simulink model "asg2_3k04"  (R2019a)
settings: Solver=FixedStepAuto  StartTime=0.0  StopTime=100  FixedStep=1E-3  RelTol=1e-3
undefined symbols (not defined in the file): D0, D1, D10, D11, D12, D13, D2, D3, D4, D5, D6, D7, D8, D9, PTA0, PTA1, PTA2, PTB23, PTB9, PTC16, PTC17, PTC2, PTC3, PTC4, PTD0, PTD1, PTD2, PTD3
libraries: frdmk64flib x21
settings Model: ExtModeTrigDuration=5  Creator=junbo  LastModifiedBy=Junbo Huang
settings OptimizationCC: EnhancedBackFolding=on  PassReuseOutputArgsAs=Individual arguments  MaxStackSize=64  OptimizeBlockOrder=speed  DifferentSizesBufferReuse=on  OptimizationCustomize=off
settings DebuggingCC: ParameterTunabilityLossMsg=error
settings HardwareCC: ProdBitPerPointer=32  ProdBitPerSizeT=32  ProdBitPerPtrDiffT=32  ProdLargestAtomicInteger=Long  ProdLargestAtomicFloat=Double  ProdWordSize=32  ProdHWDeviceType=ARM Compatible->ARM Cortex
settings SFSimCC: MATLABDynamicMemAlloc=off
settings RTWCC: SystemTargetFile=ert.tlc  HardwareBoard=NXP FRDM-K64F  TLCOptions="-aInlineSetEventsForThisBaseRateFcn=TLC_FALSE -aSuppressMultiTaskScheduler=TLC_FALSE  -aRateBasedStepFcn=0"  TemplateMakefile=ert_default_tmf  GenerateReport=on  Toolchain=GNU Tools for ARM Embedded Processors  IncludeHyperlinkInReport=on  LaunchReport=on  GenerateTraceInfo=on  GenerateTraceReport=on  GenerateTraceReportSl=on  GenerateTraceReportSf=on  GenerateTraceReportEml=on
settings CodeAppCC: ForceParamTrailComments=on  IgnoreCustomStorageClasses=off  OperatorAnnotations=on  SimulinkDataObjDesc=on  SFDataObjDesc=on  InsertBlockDesc=on
settings ERTTargetCC: SupportContinuousTime=on

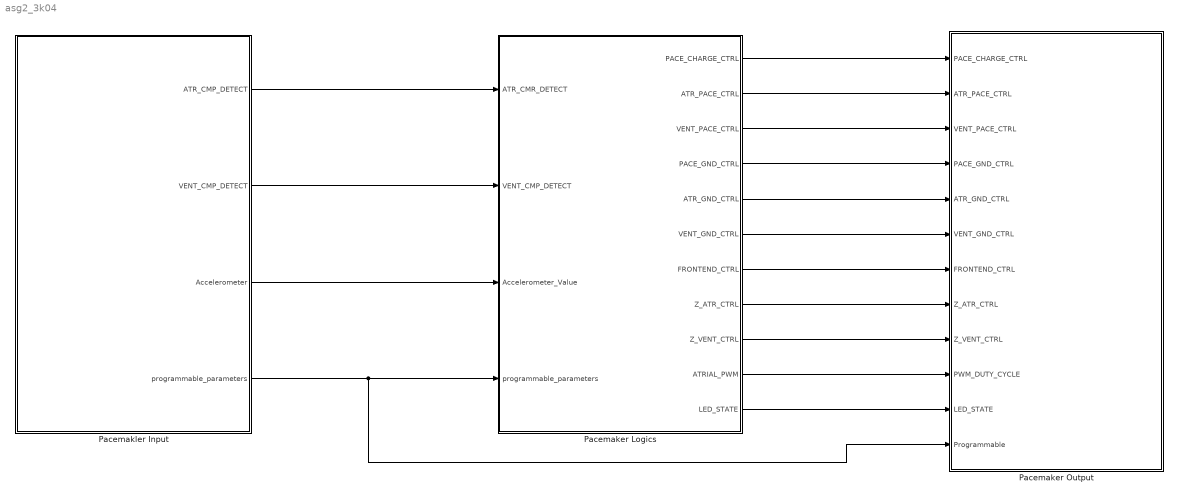
== system asg2_3k04 ==
  Pacemaker Logics : Subsystem
  Pacemaker Output : Subsystem
  Pacemakler Input : Subsystem
  wires:
  Pacemakler Input/3("Accelerometer ") -> Pacemaker Logics/3(Accelerometer_Value)
  Pacemaker Logics/11(LED_STATE) -> Pacemaker Output/11(LED_STATE)
  Pacemaker Logics/10(ATRIAL_PWM) -> Pacemaker Output/10(PWM_DUTY_CYCLE)
  Pacemaker Logics/4(PACE_GND_CTRL) -> Pacemaker Output/4(PACE_GND_CTRL)
  Pacemakler Input/1(ATR_CMP_DETECT) -> Pacemaker Logics/1(ATR_CMR_DETECT)
  Pacemaker Logics/6(VENT_GND_CTRL) -> Pacemaker Output/6(VENT_GND_CTRL)
  Pacemaker Logics/9(Z_VENT_CTRL) -> Pacemaker Output/9(Z_VENT_CTRL)
  Pacemaker Logics/8(Z_ATR_CTRL) -> Pacemaker Output/8(Z_ATR_CTRL)
  Pacemaker Logics/2(ATR_PACE_CTRL) -> Pacemaker Output/2(ATR_PACE_CTRL)
  Pacemaker Logics/3(VENT_PACE_CTRL) -> Pacemaker Output/3(VENT_PACE_CTRL)
  Pacemakler Input/2(VENT_CMP_DETECT) -> Pacemaker Logics/2(VENT_CMP_DETECT)
  Pacemaker Logics/5(ATR_GND_CTRL) -> Pacemaker Output/5(ATR_GND_CTRL)
  Pacemaker Logics/1(PACE_CHARGE_CTRL) -> Pacemaker Output/1(PACE_CHARGE_CTRL)
  Pacemakler Input/4(programmable_parameters) -> Pacemaker Output/12("Programmable "), Pacemaker Logics/4(programmable_parameters)
  Pacemaker Logics/7(FRONTEND_CTRL) -> Pacemaker Output/7(FRONTEND_CTRL)

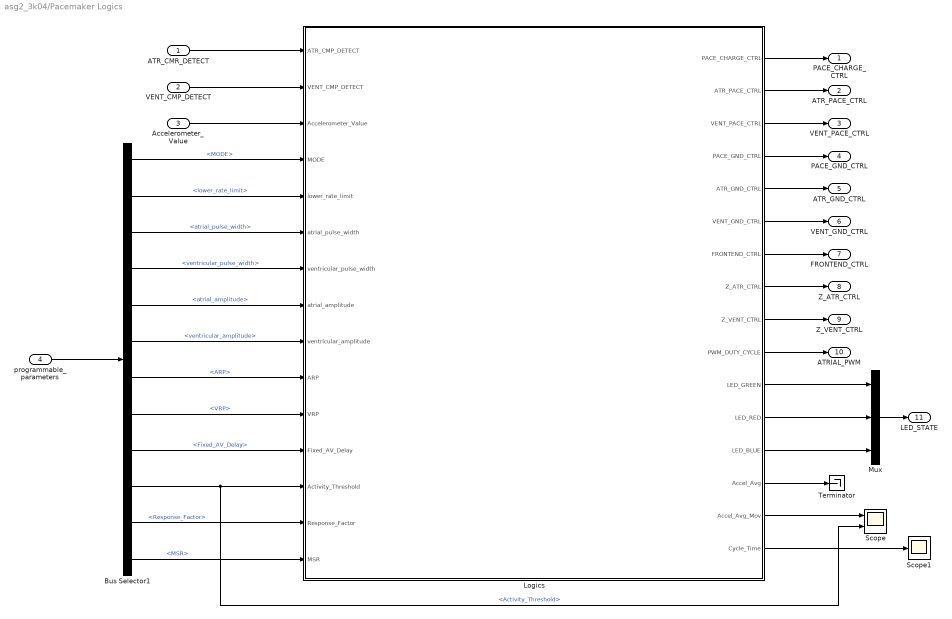
== system asg2_3k04/Pacemaker Logics ==
  ATR_CMR_DETECT : Inport
  VENT_CMP_DETECT : Inport  Port=2
  Accelerometer_Value : Inport  Port=3
  programmable_parameters : Inport  Port=4
  Bus Selector1 : BusSelector  OutputSignals=MODE,lower_rate_limit,atrial_pulse_width,ventricular_pulse_width,atrial_amplitude,ventricular_amplitude,ARP,VRP,Fixed_AV_Delay,Activity_Threshold,Response_Factor,MSR
  Logics : Stateflow chart  TreatAsAtomicUnit=on
  Mux : Mux  Inputs=3
  Scope : Scope  NumInputPorts=2
  Scope1 : Scope
  Terminator : Terminator
  PACE_CHARGE_CTRL : Outport
  ATR_PACE_CTRL : Outport  Port=2
  VENT_PACE_CTRL : Outport  Port=3
  PACE_GND_CTRL : Outport  Port=4
  ATR_GND_CTRL : Outport  Port=5
  VENT_GND_CTRL : Outport  Port=6
  FRONTEND_CTRL : Outport  Port=7
  Z_ATR_CTRL : Outport  Port=8
  Z_VENT_CTRL : Outport  Port=9
  ATRIAL_PWM : Outport  Port=10
  LED_STATE : Outport  Port=11
  wires:
  Logics/1(PACE_CHARGE_CTRL) -> PACE_CHARGE_CTRL/1
  Bus Selector1/7 -> Logics/10(ARP)  "<ARP>"
  Bus Selector1/8 -> Logics/11(VRP)  "<VRP>"
  Bus Selector1/4 -> Logics/7(ventricular_pulse_width)  "<ventricular_pulse_width>"
  Logics/2(ATR_PACE_CTRL) -> ATR_PACE_CTRL/1
  Bus Selector1/6 -> Logics/9(ventricular_amplitude)  "<ventricular_amplitude>"
  Bus Selector1/5 -> Logics/8(atrial_amplitude)  "<atrial_amplitude>"
  Bus Selector1/2 -> Logics/5(lower_rate_limit)  "<lower_rate_limit>"
  Logics/9(Z_VENT_CTRL) -> Z_VENT_CTRL/1
  Logics/8(Z_ATR_CTRL) -> Z_ATR_CTRL/1
  Logics/7(FRONTEND_CTRL) -> FRONTEND_CTRL/1
  programmable_parameters/1 -> Bus Selector1/1
  Bus Selector1/1 -> Logics/4(MODE)  "<MODE>"
  Bus Selector1/3 -> Logics/6(atrial_pulse_width)  "<atrial_pulse_width>"
  VENT_CMP_DETECT/1 -> Logics/2(VENT_CMP_DETECT)
  Logics/4(PACE_GND_CTRL) -> PACE_GND_CTRL/1
  Logics/5(ATR_GND_CTRL) -> ATR_GND_CTRL/1
  Logics/6(VENT_GND_CTRL) -> VENT_GND_CTRL/1
  ATR_CMR_DETECT/1 -> Logics/1(ATR_CMP_DETECT)
  Logics/3(VENT_PACE_CTRL) -> VENT_PACE_CTRL/1
  Logics/10(PWM_DUTY_CYCLE) -> ATRIAL_PWM/1
  Bus Selector1/9 -> Logics/12(Fixed_AV_Delay)  "<Fixed_AV_Delay>"
  Accelerometer_Value/1 -> Logics/3(Accelerometer_Value)
  Logics/11(LED_GREEN) -> Mux/1
  Logics/12(LED_RED) -> Mux/2
  Logics/13(LED_BLUE) -> Mux/3
  Mux/1 -> LED_STATE/1
  Bus Selector1/10 -> Scope/2, Logics/13(Activity_Threshold)  "<Activity_Threshold>"
  Bus Selector1/11 -> Logics/14(Response_Factor)  "<Response_Factor>"
  Bus Selector1/12 -> Logics/15(MSR)  "<MSR>"
  Logics/14(Accel_Avg) -> Terminator/1
  Logics/15(Accel_Avg_Mov) -> Scope/1
  Logics/16(Cycle_Time) -> Scope1/1

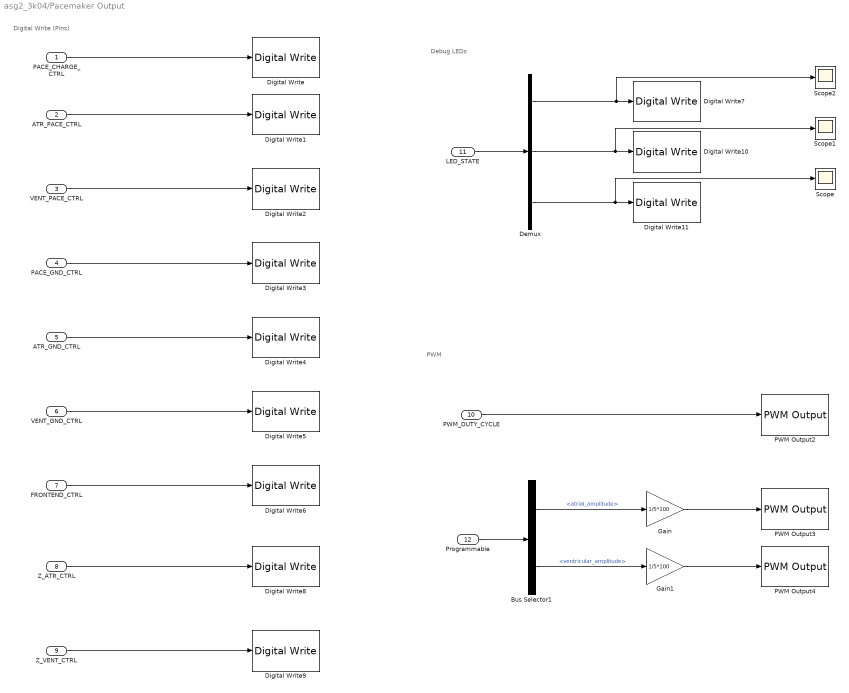
== system asg2_3k04/Pacemaker Output ==
  note: Digital Write (Pins)
  note: PWM
  note: Debug LEDs
  PACE_CHARGE_CTRL : Inport
  ATR_PACE_CTRL : Inport  Port=2
  VENT_PACE_CTRL : Inport  Port=3
  PACE_GND_CTRL : Inport  Port=4
  ATR_GND_CTRL : Inport  Port=5
  VENT_GND_CTRL : Inport  Port=6
  FRONTEND_CTRL : Inport  Port=7
  Z_ATR_CTRL : Inport  Port=8
  Z_VENT_CTRL : Inport  Port=9
  PWM_DUTY_CYCLE : Inport  Port=10
  LED_STATE : Inport  Port=11
  "Programmable " : Inport  Port=12
  Bus Selector1 : BusSelector  OutputSignals=atrial_amplitude,ventricular_amplitude
  Demux : Demux  Outputs=3
  Digital Write : frdmk64flib/Digital Write  Whichpin=PTB9 (D2)
      settings: SourceProductName=Simulink Coder Support Package for NXP FRDM-K64F Board
  Digital Write1 : frdmk64flib/Digital Write  Whichpin=PTA0 (D8)
      settings: SourceProductName=Simulink Coder Support Package for NXP FRDM-K64F Board
  Digital Write10 : frdmk64flib/Digital Write  Whichpin=RED_LED
      settings: SourceProductName=Simulink Coder Support Package for NXP FRDM-K64F Board
  Digital Write11 : frdmk64flib/Digital Write  Whichpin=BLUE_LED
      settings: SourceProductName=Simulink Coder Support Package for NXP FRDM-K64F Board
  Digital Write2 : frdmk64flib/Digital Write  Whichpin=PTC4 (D9)
      settings: SourceProductName=Simulink Coder Support Package for NXP FRDM-K64F Board
  Digital Write3 : frdmk64flib/Digital Write  Whichpin=PTD0 (D10)
      settings: SourceProductName=Simulink Coder Support Package for NXP FRDM-K64F Board
  Digital Write4 : frdmk64flib/Digital Write  Whichpin=PTD2 (D11)
      settings: SourceProductName=Simulink Coder Support Package for NXP FRDM-K64F Board
  Digital Write5 : frdmk64flib/Digital Write  Whichpin=PTD3 (D12)
      settings: SourceProductName=Simulink Coder Support Package for NXP FRDM-K64F Board
  Digital Write6 : frdmk64flib/Digital Write  Whichpin=PTD1 (D13)
      settings: SourceProductName=Simulink Coder Support Package for NXP FRDM-K64F Board
  Digital Write7 : frdmk64flib/Digital Write  Whichpin=GREEN_LED
      settings: SourceProductName=Simulink Coder Support Package for NXP FRDM-K64F Board
  Digital Write8 : frdmk64flib/Digital Write  Whichpin=PTB23 (D4)
      settings: SourceProductName=Simulink Coder Support Package for NXP FRDM-K64F Board
  Digital Write9 : frdmk64flib/Digital Write  Whichpin=PTC3 (D7)
      settings: SourceProductName=Simulink Coder Support Package for NXP FRDM-K64F Board
  Gain : Gain  Gain=1/5*100
  Gain1 : Gain  Gain=1/5*100
  PWM Output2 : frdmk64flib/PWM Output  Whichpin=PTA2 (D5)  InitialFrequency=2000  InitialDutyCycle=0
      settings: SourceProductName=Simulink Coder Support Package for NXP FRDM-K64F Board
  PWM Output3 : frdmk64flib/PWM Output  Whichpin=PTC2 (D6)  InitialFrequency=2000  InitialDutyCycle=0
      settings: SourceProductName=Simulink Coder Support Package for NXP FRDM-K64F Board
  PWM Output4 : frdmk64flib/PWM Output  Whichpin=PTA1 (D3)  InitialFrequency=2000  InitialDutyCycle=0
      settings: SourceProductName=Simulink Coder Support Package for NXP FRDM-K64F Board
  Scope : Scope
  Scope1 : Scope
  Scope2 : Scope
  wires:
  PACE_CHARGE_CTRL/1 -> Digital Write/1
  FRONTEND_CTRL/1 -> Digital Write6/1
  ATR_PACE_CTRL/1 -> Digital Write1/1
  VENT_PACE_CTRL/1 -> Digital Write2/1
  PACE_GND_CTRL/1 -> Digital Write3/1
  ATR_GND_CTRL/1 -> Digital Write4/1
  VENT_GND_CTRL/1 -> Digital Write5/1
  Z_ATR_CTRL/1 -> Digital Write8/1
  Z_VENT_CTRL/1 -> Digital Write9/1
  Bus Selector1/1 -> Gain/1  "<atrial_amplitude>"
  Bus Selector1/2 -> Gain1/1  "<ventricular_amplitude>"
  "Programmable "/1 -> Bus Selector1/1
  PWM_DUTY_CYCLE/1 -> PWM Output2/1
  Gain/1 -> PWM Output3/1
  Gain1/1 -> PWM Output4/1
  Demux/3 -> Scope/1, Digital Write11/1
  LED_STATE/1 -> Demux/1
  Demux/1 -> Scope2/1, Digital Write7/1
  Demux/2 -> Scope1/1, Digital Write10/1

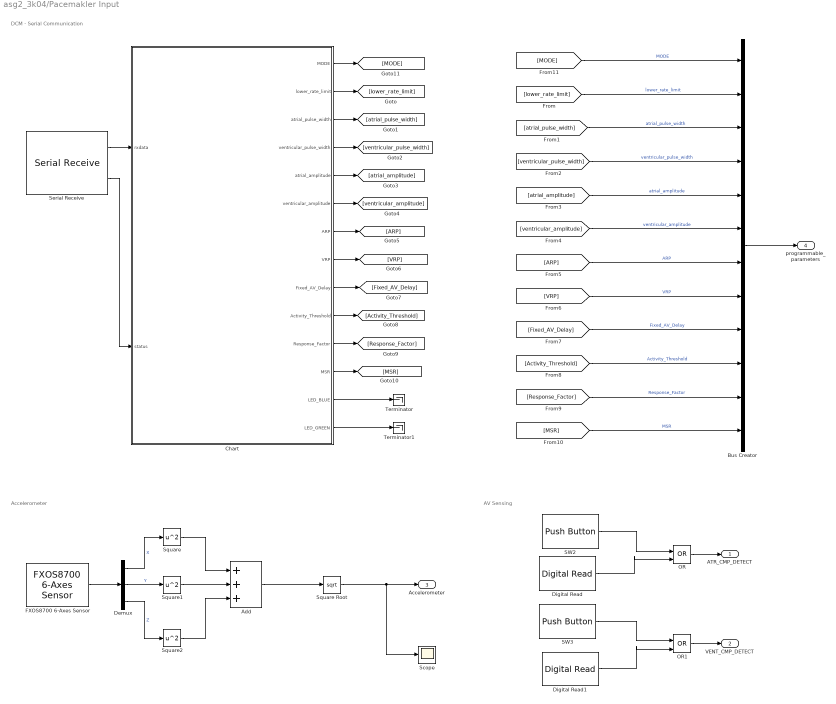
== system asg2_3k04/Pacemakler Input ==
  note: DCM - Serial Communication
  note: Accelerometer
  note: AV Sensing
  Add : Sum  Inputs=+++
  Bus Creator : BusCreator  Inputs=12
  Chart : Stateflow chart  BlockKeywords=__PRM__SERIALIZED__DATA__:Stateflow Chart,Stateflow Diagram  TreatAsAtomicUnit=on
  Demux : Demux  Outputs=3
  Digital Read : frdmk64flib/Digital Read  Whichpin=PTC16 (D0)  SampleTime=-1
      settings: SourceProductName=Simulink Coder Support Package for NXP FRDM-K64F Board
  Digital Read1 : frdmk64flib/Digital Read  Whichpin=PTC17 (D1)  SampleTime=-1
      settings: SourceProductName=Simulink Coder Support Package for NXP FRDM-K64F Board
  FXOS8700 6-Axes Sensor : frdmk64flib/FXOS8700 6-Axes Sensor  Activesensor=Accelerometer only  ODR=800Hz  HybridODR=400Hz  Accelfullrange=-4g to +4g  SampleTime=-1
      settings: SourceProductName=Simulink Coder Support Package for NXP FRDM-K64F Board
  OR : Logic  Operator=OR  IconShape=distinctive  AllPortsSameDT=off  OutDataTypeStr=boolean
  OR1 : Logic  Operator=OR  IconShape=distinctive  AllPortsSameDT=off  OutDataTypeStr=boolean
  SW2 : frdmk64flib/Push Button  Whichswitch=SW2  SampleTime1=-1
      settings: SourceProductName=Simulink Coder Support Package for NXP FRDM-K64F Board
  SW3 : frdmk64flib/Push Button  Whichswitch=SW3  SampleTime1=-1
      settings: SourceProductName=Simulink Coder Support Package for NXP FRDM-K64F Board
  Scope : Scope
  Serial Receive : frdmk64flib/Serial Receive  SCIModule=0  Baudrate=uint32(9600)  Parity=None  StopBits=1  HardwareFlowControl=None  ByteOrder=LittleEndian  DataType=uint8  DataLength=52  BlockingMode=off  OutputStatus=on  SampleTime=-1
      settings: SourceProductName=Simulink Coder Support Package for NXP FRDM-K64F Board
  Square : Math  Operator=square  SaturateOnIntegerOverflow=on
  Square Root : Sqrt  SaturateOnIntegerOverflow=on
  Square1 : Math  Operator=square  SaturateOnIntegerOverflow=on
  Square2 : Math  Operator=square  SaturateOnIntegerOverflow=on
  Terminator : Terminator
  Terminator1 : Terminator
  ATR_CMP_DETECT : Outport
  VENT_CMP_DETECT : Outport  Port=2
  "Accelerometer " : Outport  Port=3
  programmable_parameters : Outport  Port=4
  wires:
  OR/1 -> ATR_CMP_DETECT/1
  SW2/1 -> OR/1
  OR1/1 -> VENT_CMP_DETECT/1
  SW3/1 -> OR1/1
  Bus Creator/1 -> programmable_parameters/1
  [lower_rate_limit] -> Bus Creator/2  "lower_rate_limit"
  [atrial_pulse_width] -> Bus Creator/3  "atrial_pulse_width"
  [ventricular_pulse_width] -> Bus Creator/4  "ventricular_pulse_width"
  [VRP] -> Bus Creator/8  "VRP"
  [ARP] -> Bus Creator/7  "ARP"
  [atrial_amplitude] -> Bus Creator/5  "atrial_amplitude"
  [ventricular_amplitude] -> Bus Creator/6  "ventricular_amplitude"
  [Fixed_AV_Delay] -> Bus Creator/9  "Fixed_AV_Delay"
  FXOS8700 6-Axes Sensor/1 -> Demux/1
  Demux/1 -> Square/1  "X"
  Demux/2 -> Square1/1  "Y"
  Demux/3 -> Square2/1  "Z"
  Square/1 -> Add/1
  Square1/1 -> Add/2
  Square2/1 -> Add/3
  Add/1 -> Square Root/1
  [Activity_Threshold] -> Bus Creator/10  "Activity_Threshold"
  [Response_Factor] -> Bus Creator/11  "Response_Factor"
  [MSR] -> Bus Creator/12  "MSR"
  Square Root/1 -> Scope/1, "Accelerometer "/1
  [MODE] -> Bus Creator/1  "MODE"
  Chart/2(lower_rate_limit) -> [lower_rate_limit]
  Chart/3(atrial_pulse_width) -> [atrial_pulse_width]
  Chart/4(ventricular_pulse_width) -> [ventricular_pulse_width]
  Chart/5(atrial_amplitude) -> [atrial_amplitude]
  Chart/6(ventricular_amplitude) -> [ventricular_amplitude]
  Chart/7(ARP) -> [ARP]
  Chart/8(VRP) -> [VRP]
  Chart/9(Fixed_AV_Delay) -> [Fixed_AV_Delay]
  Chart/10(Activity_Threshold) -> [Activity_Threshold]
  Chart/11(Response_Factor) -> [Response_Factor]
  Chart/12(MSR) -> [MSR]
  Chart/1(MODE) -> [MODE]
  Chart/13(LED_BLUE) -> Terminator/1
  Chart/14(LED_GREEN) -> Terminator1/1
  Digital Read1/1 -> OR1/2
  Digital Read/1 -> OR/2
  Serial Receive/1 -> Chart/1(rxdata)
  Serial Receive/2 -> Chart/2(status)

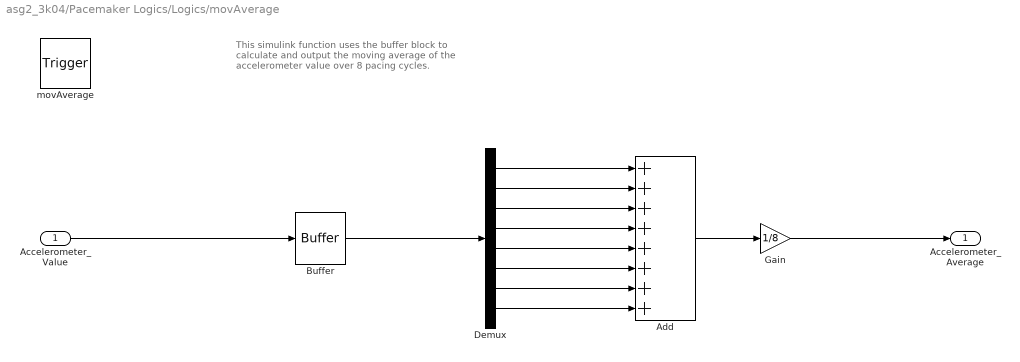
== system asg2_3k04/Pacemaker Logics/Logics/movAverage ==
  note: This simulink function uses the buffer block to calculate and output the moving average of the accelerometer value over 8 pacing cycles.
  Accelerometer_Value : Inport  OutDataTypeStr=double  PortDimensions=1
  "movAverage " : TriggerPort  TriggerType=function-call  VariantControl=(inherit)
      settings: CopyFcn=Stateflow.SLINSF.SimulinkMan.removeBlockPreDeleteFcn  PreDeleteFcn=Stateflow.SLINSF.SimulinkMan.unsafePredeleteFcn
  Add : Sum  Inputs=++++++++
  Buffer : Buffer  N=8  V=7  ic=1  OutputFrames=off
  Demux : Demux  Outputs=8
  Gain : Gain  Gain=1/8
  Accelerometer_Average : Outport  PortDimensions=1
  wires:
  Accelerometer_Value/1 -> Buffer/1
  Buffer/1 -> Demux/1
  Demux/1 -> Add/1
  Demux/2 -> Add/2
  Demux/3 -> Add/3
  Demux/4 -> Add/4
  Demux/5 -> Add/5
  Add/1 -> Gain/1
  Gain/1 -> Accelerometer_Average/1
  Demux/6 -> Add/6
  Demux/7 -> Add/7
  Demux/8 -> Add/8

== stateflow chart asg2_3k04/Pacemakler Input/Chart ==
  note: Data are unpacked and written to
      | the simulink variables as inputs.
  state Update
    entry:
    LED_BLUE = 0;
    LED_GREEN = 0;
    MODE = typecast(rxdata(3:4), 'uint16');
    %%%%
    lower_rate_limit = typecast(rxdata(5:8), 'single');
    %upper_rate_limit = typecast(rxdata(9:12), 'single');
    MSR = typecast(rxdata(13:16), 'single');
    Fixed_AV_Delay = typecast(rxdata(17:20), 'single');
    %%%%
    atrial_amplitude = typecast(rxdata(21:24), 'single');
    ventricular_amplitude = typecast(rxdata(25:28), 'single');
    atrial_pulse_width = typecast(rxdata(29:32), 'single');
    ventricular_pulse_width = typecast(rxdata(33:36), 'single');
    %%%%
    VRP = typecast(rxdata(37:40), 'single');
    ARP = typecast(rxdata(41:44), 'single');
    Activity_Threshold = typecast(rxdata(45:48), 'single');
    Response_Factor = typecast(rxdata(49:52), 'single');
  state Init
    entry:
    MODE= 5;
    lower_rate_limit=60;
    atrial_pulse_width=20;
    ventricular_pulse_width=20;
    atrial_amplitude=3;
    ventricular_amplitude=3;
    ARP=150;
    VRP=150;
    Fixed_AV_Delay=20;
    Activity_Threshold=1.5;
    Response_Factor=1;
    MSR = 120;
    LED_GREEN = 0;
    LED_BLUE = 0;
    %%%%%%Initialize Parameters%%%%%%%%
  state StandBy
    entry:
    LED_BLUE = 0;
    LED_GREEN = 0;
  note: Check if serial
      | com succeed
  note: Check the first byte of
      | Serial Data
  note: We set the first byte to 1 in
      | DCM and an acknowledgement
      | for the begin of packed serial data
  (default) -> Init
  Update -> StandBy : after(500, msec)
  (junction 42) -> StandBy [order 2]
  Init -> StandBy
  StandBy -> (junction 42) : [status == 0]
  (junction 42) -> Update [order 1] : [rxdata(1) == hex2dec('1') ]
  data: MODE output uint16; rxdata input uint8; status input uint8; lower_rate_limit output single; atrial_pulse_width output single; ventricular_pulse_width output single; atrial_amplitude output single; ventricular_amplitude output single; ARP output single; VRP output single; Fixed_AV_Delay output single; Activity_Threshold output single; Response_Factor output single; MSR output single; LED_BLUE output uint8; LED_GREEN output uint8

== stateflow chart asg2_3k04/Pacemaker Logics/Logics ==
  state VOO_MODE
    note: Charge up C22 and discharge C21 to ground
    note: Discharge C22 to C21 which charge up C21
    state VOO_CHARGE
      entry:
      PACE_CHARGE_CTRL = true;
      VENT_PACE_CTRL = false;
      VENT_GND_CTRL = true;
      PACE_GND_CTRL = true;
      Z_ATR_CTRL = false;
      Z_VENT_CTRL = false;
      Cycle_Time = (60/lower_rate_limit)*1000;
      LED_GREEN = 0;
    state VOO_PACE
      entry:
      PACE_CHARGE_CTRL = false;
      VENT_PACE_CTRL = true;
      VENT_GND_CTRL = false;
      PACE_GND_CTRL = true;
      Z_ATR_CTRL = false;
      Z_VENT_CTRL = false;
      PWM_DUTY_CYCLE = (ventricular_amplitude/5)*100;
      LED_GREEN = 1;
    VOO_MODE.VOO_CHARGE -> VOO_MODE.VOO_PACE [order 2] : after(Cycle_Time - ventricular_pulse_width,msec)
    VOO_MODE.VOO_PACE -> VOO_MODE.VOO_CHARGE : after(ventricular_pulse_width,msec)
  state VOOR_MODE
    state PACE [parallel]
      settings: executionOrder=1
      note: Charge up C22 and discharge C21 to ground
      note: Discharge C22 to C21 which charge up C21
      state VOO_CHARGE
        entry:
        PACE_CHARGE_CTRL = true;
        VENT_PACE_CTRL = false;
        VENT_GND_CTRL = true;
        PACE_GND_CTRL = true;
        Z_ATR_CTRL = false;
        Z_VENT_CTRL = false;
        LED_GREEN = 0;
        Accel_Avg_Mov = movAverage(Accel_Avg);
        Cycle_Time = rateConversion(lower_rate_limit, MSR, Response_Factor, Activity_Threshold, Accel_Avg_Mov);
      state VOO_PACE
        entry:
        PACE_CHARGE_CTRL = false;
        VENT_PACE_CTRL = true;
        VENT_GND_CTRL = false;
        PACE_GND_CTRL = true;
        Z_ATR_CTRL = false;
        Z_VENT_CTRL = false;
        PWM_DUTY_CYCLE = (ventricular_amplitude/5)*100;
        LED_GREEN = 1;
      VOOR_MODE.PACE.VOO_CHARGE -> VOOR_MODE.PACE.VOO_PACE [order 1] : after(Cycle_Time - ventricular_pulse_width,msec)
      (default) -> VOOR_MODE.PACE.VOO_CHARGE
      VOOR_MODE.PACE.VOO_PACE -> VOOR_MODE.PACE.VOO_CHARGE : after(ventricular_pulse_width,msec)
    state RateAdaptive [parallel]
      settings: executionOrder=2
      state Update_Acc_Avg
        entry:
        [Accel_Avg, Cycle_Counter] = average(Accel_Val_Vec, Cycle_Counter);
      state Store_Acc_Val
        entry:
        [Accel_Val_Vec, Cycle_Counter] = storeSamples(Accelerometer_Value, Accel_Val_Vec, Cycle_Counter);
      VOOR_MODE.RateAdaptive.Store_Acc_Val -> VOOR_MODE.RateAdaptive.Update_Acc_Avg [order 1] : [Cycle_Counter >= 500]
      VOOR_MODE.RateAdaptive.Update_Acc_Avg -> VOOR_MODE.RateAdaptive.Store_Acc_Val
      (default) -> VOOR_MODE.RateAdaptive.Store_Acc_Val
      VOOR_MODE.RateAdaptive.Store_Acc_Val -> VOOR_MODE.RateAdaptive.Store_Acc_Val [order 2]
  state Accelerometer_Average = movAverage(Accelerometer_Value) [function]
  note: Starting state, open all the switchs for safety
  state Initialize
    entry:
    Cycle_Time = (60/lower_rate_limit)*1000;
    Accel_Val_Vec = ones(500,1);
    Accel_Avg = 1;
    Accel_Avg_Mov = 1;
    Cycle_Counter = 0;
  note: VOO Mode
  state AOO_MODE
    note: Charge up C22 and discharge C21 to ground
    note: Discharge C22 to C21 which charge up C21
    state AOO_CHARGE
      entry:
      PACE_CHARGE_CTRL = true;
      %charge C22
      ATR_PACE_CTRL = false;
      ATR_GND_CTRL = true;
      PACE_GND_CTRL = true;
      %discharge C21
      Z_ATR_CTRL = false;
      Z_VENT_CTRL = false;
      Cycle_Time = (60/lower_rate_limit)*1000;
      LED_RED = 0;
    state AOO_PACE
      entry:
      PACE_CHARGE_CTRL = false;
      PACE_GND_CTRL = true; %charge C21
      ATR_PACE_CTRL = true; %discharge C22
      ATR_GND_CTRL = false;
      Z_ATR_CTRL = false;
      Z_VENT_CTRL = false;
      PWM_DUTY_CYCLE = (atrial_amplitude/5)*100;
      %set PWM duty cycle based on input amplitude
      LED_RED = 1;
    note: Lower rate limit is converted to period of cycle
    note: Pace for the period specified by pulse width
    AOO_MODE.AOO_CHARGE -> AOO_MODE.AOO_PACE [order 1] : after(Cycle_Time - atrial_pulse_width,msec)
    AOO_MODE.AOO_PACE -> AOO_MODE.AOO_CHARGE : after(atrial_pulse_width,msec)
  state AOOR_MODE
    state Pace [parallel]
      settings: executionOrder=1
      note: Charge up C22 and discharge C21 to ground
      note: Discharge C22 to C21 which charge up C21
      state AOO_CHARGE
        entry:
        PACE_CHARGE_CTRL = true;
        %charge C22
        ATR_PACE_CTRL = false;
        ATR_GND_CTRL = true;
        PACE_GND_CTRL = true;
        %discharge C21
        Z_ATR_CTRL = false;
        Z_VENT_CTRL = false;
        LED_RED = 0;
        Accel_Avg_Mov = movAverage(Accel_Avg);
        Cycle_Time = rateConversion(lower_rate_limit, MSR, Response_Factor, Activity_Threshold, Accel_Avg_Mov);
      state AOO_PACE
        entry:
        PACE_CHARGE_CTRL = false;
        PACE_GND_CTRL = true; %charge C21
        ATR_PACE_CTRL = true; %discharge C22
        ATR_GND_CTRL = false;
        Z_ATR_CTRL = false;
        Z_VENT_CTRL = false;
        PWM_DUTY_CYCLE = (atrial_amplitude/5)*100;
        LED_RED = 1
        %set PWM duty cycle based on input amplitude
      note: Lower rate limit is converted to period of cycle
      note: Pace for the period specified by pulse width
      AOOR_MODE.Pace.AOO_CHARGE -> AOOR_MODE.Pace.AOO_PACE [order 1] : after(Cycle_Time - atrial_pulse_width,msec)
      (default) -> AOOR_MODE.Pace.AOO_CHARGE
      AOOR_MODE.Pace.AOO_PACE -> AOOR_MODE.Pace.AOO_CHARGE : after(atrial_pulse_width,msec)
    state RateAdaptive [parallel]
      settings: executionOrder=2
      state Update_Acc_Avg
        entry:
        [Accel_Avg, Cycle_Counter] = average(Accel_Val_Vec, Cycle_Counter);
      state Store_Acc_Val
        entry:
        [Accel_Val_Vec, Cycle_Counter] = storeSamples(Accelerometer_Value, Accel_Val_Vec, Cycle_Counter);
      AOOR_MODE.RateAdaptive.Store_Acc_Val -> AOOR_MODE.RateAdaptive.Update_Acc_Avg [order 1] : [Cycle_Counter >= 500]
      AOOR_MODE.RateAdaptive.Update_Acc_Avg -> AOOR_MODE.RateAdaptive.Store_Acc_Val
      (default) -> AOOR_MODE.RateAdaptive.Store_Acc_Val
      AOOR_MODE.RateAdaptive.Store_Acc_Val -> AOOR_MODE.RateAdaptive.Store_Acc_Val [order 2]
  state MAIN
    entry:
    PACE_CHARGE_CTRL = false;
    VENT_PACE_CTRL = false;
    ATR_PACE_CTRL = false;
    VENT_GND_CTRL = false;
    ATR_GND_CTRL = false;
    PACE_GND_CTRL = false;
    FRONTEND_CTRL = false;
    Z_ATR_CTRL = false;
    Z_VENT_CTRL = false;
    %%% Initialize LEDs
    LED_GREEN = 0;
    LED_RED = 0;
    LED_BLUE = 0;
  note: AOO Mode
  note: MODE
      | Mode Name
      |
      | 0
      | VOO
      |
      | 1
      | AOO
      |
      | 2
      | VVI
      |
      | 3
      | AAI
      |
      | 4
      | DOO
      |
      | 5
      | VOOR
      |
      | 6
      | AOOR
      |
      | 7
      | VVIR
      |
      | 8
      | AAIR
      |
      | 9
      | DOOR
  note: VVI Mode
  state VVI_MODE
    note: Charge up C22 and discharge C21 to ground, sensing natrual signal
    note: Discharge C22 to C21 which charge up C21
    state VVI_CHARGE
      entry:
      FRONTEND_CTRL = true;
      PACE_CHARGE_CTRL = true;
      VENT_PACE_CTRL = false;
      VENT_GND_CTRL = true;
      PACE_GND_CTRL = true;
      Z_ATR_CTRL = false;
      Z_VENT_CTRL = false;
      Cycle_Time = (60/lower_rate_limit)*1000;
    state VVI_PACE
      entry:
      PACE_CHARGE_CTRL = false;
      VENT_PACE_CTRL = true;
      VENT_GND_CTRL = false;
      PACE_GND_CTRL = true;
      Z_ATR_CTRL = false;
      Z_VENT_CTRL = false;
      PWM_DUTY_CYCLE =  (ventricular_amplitude/5)*100;
      LED_GREEN = 1;
    note: Signal detected, refresh VRP counting
    state VVI_DETECTED
      FRONTEND_CTRL = false;
      %stay in this state during the ...
      %refractory period
      PACE_CHARGE_CTRL = true;
      VENT_PACE_CTRL = false;
      VENT_GND_CTRL = true;
      PACE_GND_CTRL = true;
      Z_ATR_CTRL = false;
      Z_VENT_CTRL = false;
      LED_GREEN = 0;
    note: Inhibit
    note: Refractory Period
    VVI_MODE.VVI_CHARGE -> VVI_MODE.VVI_PACE [order 3] : after(Cycle_Time - VRP - ventricular_pulse_width,msec)
    VVI_MODE.VVI_PACE -> VVI_MODE.VVI_DETECTED : after(ventricular_pulse_width,msec)
    VVI_MODE.VVI_DETECTED -> VVI_MODE.VVI_CHARGE : after(VRP, msec)
    VVI_MODE.VVI_CHARGE -> (junction 125) [order 2] : [VENT_CMP_DETECT == true]
    (junction 125) -> VVI_MODE.VVI_DETECTED : after(ventricular_pulse_width, msec)
  state VVIR_MODE
    state PACE [parallel]
      settings: executionOrder=1
      note: Charge up C22 and discharge C21 to ground, sensing natrual signal
      note: Discharge C22 to C21 which charge up C21
      state VVI_CHARGE
        entry:
        FRONTEND_CTRL = true;
        PACE_CHARGE_CTRL = true;
        VENT_PACE_CTRL = false;
        VENT_GND_CTRL = true;
        PACE_GND_CTRL = true;
        Z_ATR_CTRL = false;
        Z_VENT_CTRL = false;
        Accel_Avg_Mov = movAverage(Accel_Avg);
        Cycle_Time = rateConversion(lower_rate_limit, MSR, Response_Factor, Activity_Threshold, Accel_Avg_Mov);
      state VVI_PACE
        entry:
        PACE_CHARGE_CTRL = false;
        VENT_PACE_CTRL = true;
        VENT_GND_CTRL = false;
        PACE_GND_CTRL = true;
        Z_ATR_CTRL = false;
        Z_VENT_CTRL = false;
        PWM_DUTY_CYCLE =  (ventricular_amplitude/5)*100;
        LED_GREEN = 1;
      note: Signal detected, refresh VRP counting
      state VVI_DETECTED
        FRONTEND_CTRL = false;
        %stay in this state during the ...
        %refractory period
        PACE_CHARGE_CTRL = true;
        VENT_PACE_CTRL = false;
        VENT_GND_CTRL = true;
        PACE_GND_CTRL = true;
        Z_ATR_CTRL = false;
        Z_VENT_CTRL = false;
        LED_GREEN = 0;
      note: Inhibit
      note: Refractory Period
      VVIR_MODE.PACE.VVI_CHARGE -> VVIR_MODE.PACE.VVI_PACE [order 2] : after(Cycle_Time - VRP - ventricular_pulse_width,msec)
      (default) -> VVIR_MODE.PACE.VVI_CHARGE
      VVIR_MODE.PACE.VVI_PACE -> VVIR_MODE.PACE.VVI_DETECTED : after(ventricular_pulse_width,msec)
      VVIR_MODE.PACE.VVI_DETECTED -> VVIR_MODE.PACE.VVI_CHARGE : after(VRP, msec)
      VVIR_MODE.PACE.VVI_CHARGE -> (junction 271) [order 1] : [VENT_CMP_DETECT == true]
      (junction 271) -> VVIR_MODE.PACE.VVI_DETECTED : after(ventricular_pulse_width, msec)
    state RateAdaptive [parallel]
      settings: executionOrder=2
      state Update_Acc_Avg
        entry:
        [Accel_Avg, Cycle_Counter] = average(Accel_Val_Vec, Cycle_Counter);
      state Store_Acc_Val
        entry:
        [Accel_Val_Vec, Cycle_Counter] = storeSamples(Accelerometer_Value, Accel_Val_Vec, Cycle_Counter);
      VVIR_MODE.RateAdaptive.Store_Acc_Val -> VVIR_MODE.RateAdaptive.Update_Acc_Avg [order 1] : [Cycle_Counter >= 500]
      VVIR_MODE.RateAdaptive.Update_Acc_Avg -> VVIR_MODE.RateAdaptive.Store_Acc_Val
      (default) -> VVIR_MODE.RateAdaptive.Store_Acc_Val
      VVIR_MODE.RateAdaptive.Store_Acc_Val -> VVIR_MODE.RateAdaptive.Store_Acc_Val [order 2]
  note: AAI Mode
  state AAIR_MODE
    state PACE [parallel]
      settings: executionOrder=1
      note: Charge up C22 and discharge C21 to ground, sensing natrual signal
      note: Discharge C22 to C21 which charge up C21
      state AAI_CHARGE
        entry:
        FRONTEND_CTRL = true;
        PACE_CHARGE_CTRL = true;
        ATR_PACE_CTRL = false;
        ATR_GND_CTRL = true;
        PACE_GND_CTRL = true;
        Z_ATR_CTRL = false;
        Z_VENT_CTRL = false;
        Accel_Avg_Mov = movAverage(Accel_Avg);
        Cycle_Time = rateConversion(lower_rate_limit, MSR, Response_Factor, Activity_Threshold, Accel_Avg_Mov);
      state AAI_PACE
        entry:
        PACE_CHARGE_CTRL = false;
        ATR_PACE_CTRL = true;
        ATR_GND_CTRL = false;
        PACE_GND_CTRL = true;
        Z_ATR_CTRL = false;
        Z_VENT_CTRL = false;
        PWM_DUTY_CYCLE = (atrial_amplitude/5)*100;
        LED_RED = 1;
      note: Signal detected, refresh ARP counting
      note: Inhibit
      state AAI_DETECTED
        FRONTEND_CTRL = false;
        %stay in this state during the ...
        %refractory period
        PACE_CHARGE_CTRL = true;
        ATR_PACE_CTRL = false;
        ATR_GND_CTRL = true;
        PACE_GND_CTRL = true;
        Z_ATR_CTRL = false;
        Z_VENT_CTRL = false;
        LED_RED = 0;
      note: Refractory Period
      AAIR_MODE.PACE.AAI_CHARGE -> AAIR_MODE.PACE.AAI_PACE [order 2] : after(Cycle_Time - ARP - atrial_pulse_width,msec)
      (default) -> AAIR_MODE.PACE.AAI_CHARGE
      AAIR_MODE.PACE.AAI_PACE -> AAIR_MODE.PACE.AAI_DETECTED : after(atrial_pulse_width,msec)
      AAIR_MODE.PACE.AAI_DETECTED -> AAIR_MODE.PACE.AAI_CHARGE : after(ARP,msec)
      AAIR_MODE.PACE.AAI_CHARGE -> (junction 245) [order 1] : [ATR_CMP_DETECT == true]
      (junction 245) -> AAIR_MODE.PACE.AAI_DETECTED : after(atrial_pulse_width, msec)
    state RateAdaptive [parallel]
      settings: executionOrder=2
      state Update_Acc_Avg
        entry:
        [Accel_Avg, Cycle_Counter] = average(Accel_Val_Vec, Cycle_Counter);
      state Store_Acc_Val
        entry:
        [Accel_Val_Vec, Cycle_Counter] = storeSamples(Accelerometer_Value, Accel_Val_Vec, Cycle_Counter);
      AAIR_MODE.RateAdaptive.Store_Acc_Val -> AAIR_MODE.RateAdaptive.Update_Acc_Avg [order 1] : [Cycle_Counter >= 500]
      AAIR_MODE.RateAdaptive.Update_Acc_Avg -> AAIR_MODE.RateAdaptive.Store_Acc_Val
      (default) -> AAIR_MODE.RateAdaptive.Store_Acc_Val
      AAIR_MODE.RateAdaptive.Store_Acc_Val -> AAIR_MODE.RateAdaptive.Store_Acc_Val [order 2]
  state AAI_MODE
    note: Charge up C22 and discharge C21 to ground, sensing natrual signal
    note: Discharge C22 to C21 which charge up C21
    state AAI_CHARGE
      entry:
      FRONTEND_CTRL = true;
      PACE_CHARGE_CTRL = true;
      ATR_PACE_CTRL = false;
      ATR_GND_CTRL = true;
      PACE_GND_CTRL = true;
      Z_ATR_CTRL = false;
      Z_VENT_CTRL = false;
      Cycle_Time = (60/lower_rate_limit)*1000;
    state AAI_PACE
      entry:
      PACE_CHARGE_CTRL = false;
      ATR_PACE_CTRL = true;
      ATR_GND_CTRL = false;
      PACE_GND_CTRL = true;
      Z_ATR_CTRL = false;
      Z_VENT_CTRL = false;
      PWM_DUTY_CYCLE = (atrial_amplitude/5)*100;
      LED_RED = 1;
    note: Signal detected, refresh ARP counting
    state AAI_DETECTED
      FRONTEND_CTRL = false;
      %stay in this state during the ...
      %refractory period
      PACE_CHARGE_CTRL = true;
      ATR_PACE_CTRL = false;
      ATR_GND_CTRL = true;
      PACE_GND_CTRL = true;
      Z_ATR_CTRL = false;
      Z_VENT_CTRL = false;
      LED_RED = 0;
    note: Inhibit
    note: Refractory Period
    AAI_MODE.AAI_CHARGE -> AAI_MODE.AAI_PACE [order 3] : after(Cycle_Time - ARP - atrial_pulse_width,msec)
    AAI_MODE.AAI_PACE -> AAI_MODE.AAI_DETECTED : after(atrial_pulse_width,msec)
    AAI_MODE.AAI_DETECTED -> AAI_MODE.AAI_CHARGE : after(ARP,msec)
    AAI_MODE.AAI_CHARGE -> (junction 139) [order 2] : [ATR_CMP_DETECT == true]
    (junction 139) -> AAI_MODE.AAI_DETECTED : after(atrial_pulse_width, msec)
  note: DOO Mode
  state DOO_MODE
    note: Charge up C22 and discharge C21 to ground
    state DOO_CHARGE
      entry:
      PACE_CHARGE_CTRL = true;
      PACE_GND_CTRL = true;
      %Turn off both
      ATR_PACE_CTRL = false;
      ATR_GND_CTRL = true;
      VENT_PACE_CTRL = false;
      VENT_GND_CTRL = true;
      %%%
      Z_ATR_CTRL = false;
      Z_VENT_CTRL = false;
      LED_BLUE = 0;
      Cycle_Time = (60/lower_rate_limit)*1000;
    note: Discharge C22 to C21 which charge up C21
    state ATRIAL_PACE
      entry:
      PACE_CHARGE_CTRL = false;
      PACE_GND_CTRL = true;
      %Pace Atrium
      ATR_PACE_CTRL = true;
      ATR_GND_CTRL = false;
      %%
      Z_ATR_CTRL = false;
      Z_VENT_CTRL = false;
      PWM_DUTY_CYCLE = (atrial_amplitude/5)*100;
      LED_BLUE = 1;
    state VENT_PACE
      entry:
      PACE_CHARGE_CTRL = false;
      PACE_GND_CTRL = true;
      %charge C21
      VENT_PACE_CTRL = true;
      VENT_GND_CTRL = false;
      Z_ATR_CTRL = false;
      Z_VENT_CTRL = false;
      PWM_DUTY_CYCLE = (ventricular_amplitude/5)*100;
      LED_BLUE = 1;
    state AV_DELAY
      entry:
      ATR_PACE_CTRL = false;
      ATR_GND_CTRL = false;
      LED_BLUE = 0;
    note: Pace Ventricle
    note: Close atrial switches
    DOO_MODE.DOO_CHARGE -> DOO_MODE.ATRIAL_PACE [order 2] : after(Cycle_Time - ventricular_pulse_width - Fixed_AV_Delay ,msec)
    DOO_MODE.ATRIAL_PACE -> AV_DELAY : after(atrial_pulse_width, msec)
    DOO_MODE.VENT_PACE -> DOO_MODE.DOO_CHARGE : after(ventricular_pulse_width, msec)
    AV_DELAY -> DOO_MODE.VENT_PACE : after(Fixed_AV_Delay - atrial_pulse_width, msec)
  state DOOR_MODE
    state PACE [parallel]
      settings: executionOrder=1
      note: Charge up C22 and discharge C21 to ground
      note: Discharge C22 to C21 which charge up C21
      state DOO_CHARGE
        entry:
        PACE_CHARGE_CTRL = true;
        PACE_GND_CTRL = true;
        %Turn off both
        ATR_PACE_CTRL = false;
        ATR_GND_CTRL = true;
        VENT_PACE_CTRL = false;
        VENT_GND_CTRL = true;
        %%%
        Z_ATR_CTRL = false;
        Z_VENT_CTRL = false;
        LED_BLUE = 0;
        Accel_Avg_Mov = movAverage(Accel_Avg);
        Cycle_Time = rateConversion(lower_rate_limit, MSR, Response_Factor, Activity_Threshold, Accel_Avg_Mov);
      state ATRIAL_PACE
        entry:
        PACE_CHARGE_CTRL = false;
        PACE_GND_CTRL = true;
        %Pace Atrium
        ATR_PACE_CTRL = true;
        ATR_GND_CTRL = false;
        %%
        Z_ATR_CTRL = false;
        Z_VENT_CTRL = false;
        PWM_DUTY_CYCLE = (atrial_amplitude/5)*100;
        LED_BLUE = 1;
      state VENT_PACE
        entry:
        PACE_CHARGE_CTRL = false;
        PACE_GND_CTRL = true;
        %charge C21
        VENT_PACE_CTRL = true;
        VENT_GND_CTRL = false;
        Z_ATR_CTRL = false;
        Z_VENT_CTRL = false;
        PWM_DUTY_CYCLE = (ventricular_amplitude/5)*100;
        LED_BLUE = 1;
      state AV_Delay
        entry:
        ATR_PACE_CTRL = false;
        ATR_GND_CTRL = false;
        LED_BLUE = 0;
      DOOR_MODE.PACE.DOO_CHARGE -> DOOR_MODE.PACE.ATRIAL_PACE [order 1] : after(Cycle_Time - ventricular_pulse_width - Fixed_AV_Delay ,msec)
      (default) -> DOOR_MODE.PACE.DOO_CHARGE
      DOOR_MODE.PACE.ATRIAL_PACE -> AV_Delay : after(atrial_pulse_width, msec)
      DOOR_MODE.PACE.VENT_PACE -> DOOR_MODE.PACE.DOO_CHARGE : after(ventricular_pulse_width, msec)
      AV_Delay -> DOOR_MODE.PACE.VENT_PACE : after(Fixed_AV_Delay - atrial_pulse_width, msec)
    state RateAdaptive [parallel]
      settings: executionOrder=2
      state Update_Acc_Avg
        entry:
        [Accel_Avg, Cycle_Counter] = average(Accel_Val_Vec, Cycle_Counter);
      state Store_Acc_Val
        entry:
        [Accel_Val_Vec, Cycle_Counter] = storeSamples(Accelerometer_Value, Accel_Val_Vec, Cycle_Counter);
      DOOR_MODE.RateAdaptive.Store_Acc_Val -> DOOR_MODE.RateAdaptive.Update_Acc_Avg [order 1] : [Cycle_Counter >= 500]
      DOOR_MODE.RateAdaptive.Update_Acc_Avg -> DOOR_MODE.RateAdaptive.Store_Acc_Val
      (default) -> DOOR_MODE.RateAdaptive.Store_Acc_Val
      DOOR_MODE.RateAdaptive.Store_Acc_Val -> DOOR_MODE.RateAdaptive.Store_Acc_Val [order 2]
  VOOR_MODE.PACE.VOO_CHARGE -> MAIN [order 2] : [MODE ~= 5]
  AOO_MODE.AOO_CHARGE -> MAIN [order 2] : [MODE ~= 1]
  VOO_MODE.VOO_CHARGE -> MAIN [order 1] : [MODE ~= 0]
  VVIR_MODE.PACE.VVI_CHARGE -> MAIN [order 3] : [MODE ~= 7]
  DOOR_MODE.PACE.DOO_CHARGE -> MAIN [order 2] : [MODE ~= 9]
  AAIR_MODE.PACE.AAI_CHARGE -> MAIN [order 3] : [MODE ~= 8]
  AOOR_MODE.Pace.AOO_CHARGE -> MAIN [order 2] : [MODE ~= 6]
  AAI_MODE.AAI_CHARGE -> MAIN [order 1] : [MODE ~= 3]
  MAIN -> VOO_MODE.VOO_CHARGE [order 1] : [MODE == 0]
  MAIN -> VOOR_MODE [order 6] : [MODE == 5]
  (default) -> Initialize
  VVI_MODE.VVI_CHARGE -> MAIN [order 1] : [MODE ~= 2]
  DOO_MODE.DOO_CHARGE -> MAIN [order 1] : [MODE ~= 4]
  Initialize -> MAIN
  MAIN -> AOOR_MODE [order 7] : [MODE == 6]
  MAIN -> AOO_MODE.AOO_CHARGE [order 2] : [MODE == 1]
  MAIN -> VVI_MODE.VVI_CHARGE [order 3] : [MODE == 2]
  MAIN -> AAI_MODE.AAI_CHARGE [order 4] : [MODE == 3]
  MAIN -> VVIR_MODE [order 8] : [MODE == 7]
  MAIN -> DOO_MODE.DOO_CHARGE [order 5] : [MODE == 4]
  MAIN -> AAIR_MODE [order 9] : [MODE == 8]
  MAIN -> DOOR_MODE [order 10] : [MODE == 9]
  data: Accelerometer_Value function_input double size=1; Accelerometer_Average function_output size=1; LRL function_input; MSR_C function_input; RF function_input; AtvThreshold function_input; AccAvg function_input; Cycle function_output; AccVal function_input; AccVector function_output; AccVector function_input; counter function_input; counter function_output; SignalVec function_input; counter function_input; acc_average function_output; counter function_output; ATR_CMP_DETECT input boolean size=1; VENT_CMP_DETECT input boolean size=1; Accelerometer_Value input size=1; PACE_CHARGE_CTRL output boolean; ATR_PACE_CTRL output boolean; VENT_PACE_CTRL output boolean; PACE_GND_CTRL output boolean; ATR_GND_CTRL output boolean; VENT_GND_CTRL output boolean; FRONTEND_CTRL output boolean; MODE input; lower_rate_limit input; atrial_pulse_width input; ventricular_pulse_width input; atrial_amplitude input; ventricular_amplitude input; ARP input; VRP input; Z_ATR_CTRL output boolean; Z_VENT_CTRL output boolean; PWM_DUTY_CYCLE output; Fixed_AV_Delay input; LED_GREEN output uint8; LED_RED output uint8; LED_BLUE output uint8; Activity_Threshold input; Response_Factor input; Accel_Avg output; Accel_Avg_Mov output; MSR input; Cycle_Time output; Accel_Val_Vec local size=500; Cycle_Counter local
  function Cycle = rateConversion(LRL, MSR_C, RF, AtvThreshold, AccAvg):
    | function Cycle = rateConversion(LRL, MSR_C, RF, AtvThreshold, AccAvg)
    |     
    |     if AccAvg < AtvThreshold %%if calculated accelerometer value less than threshold,
    |         Rate = LRL;                %%set the rate to LRL and calculate the Cycle time
    |         Cycle = (60/Rate)*1000;
    |         return;
    |     end    
    |     
    |     %%%%%%%%% rate adaptive function %%%%%%%%
    |     Delta_Y = MSR_C - LRL;
    |     RF_FACTOR = (16 - RF + 1)/16; %convert the Response factor to a gain from 1/16 to 16/16
    |     Max_Activity_Offset = 4;
    |     Min_Activity_Offset = 1;
    |     Delta_X = Min_Activity_Offset + (Max_Activity_Offset - Min_Activity_Offset)*RF_FACTOR;
    |     Slope = Delta_Y/Delta_X; %calculate slope of curve, where X-axis is Activity level and Y-axis is Rate(BPM)
    |     
    |     Rate = LRL + Slope * (AccAvg - AtvThreshold);% y = f(x), where x is AccAvg, y is Rate
    |     %%%%%%%%%%%%%%%%%%%%%
    |     
    |     if Rate >= MSR_C %%if the calculated rate is larger than Max Sensor Rate,
    |         Rate = MSR_C;%%set rate to Max Sensor Rate
    |     end
    |     
    |     Cycle = (60/Rate)*1000;%%calculate Cycle time based on rate
    |     
    | end
  function [AccVector, counter] = storeSamples(AccVal, AccVector, counter):
    | function [AccVector, counter] = storeSamples(AccVal, AccVector, counter) %%excecute on every sample time (0.001s)
    |     counter = counter + 1; %increment cycle counter
    |     AccVector(counter) = AccVal; %store current accelerometer value into a vector of size 500
    | end
  function [acc_average, counter] = average(SignalVec, counter):
    | function [acc_average, counter] = average(SignalVec, counter)
    |     acc_average = 0; % initialize acc_average
    |     
    |     for i = 1:counter % calculate the average value of accelerometer over 500 samples
    |                        %iterate through the vector created by
    |                        %storeSamples()
    |         
    |         acc_average = acc_average + SignalVec(i);
    |         
    |     end
    |     
    |     acc_average = acc_average/counter; %%calculate average
    |     counter = 0; %%reset cycle counter
    |     
    | end
